simulink model "pmdc_simulink"  (R2025b)
settings: Solver=VariableStepAuto  StartTime=0.0  StopTime=3  RelTol=1e-3
undefined symbols (not defined in the file or in its folder): Bm, J, Kv, La, Ra, TL, Va
settings Model: Creator=Seyma  LastModifiedBy=Seyma
settings DataIOCC: SaveFormat=Array  ReturnWorkspaceOutputs=off

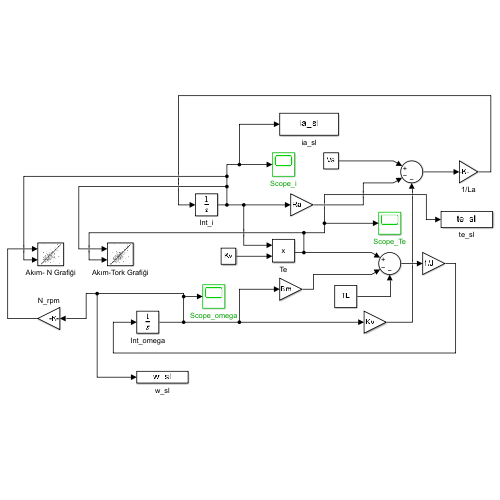
[thumbnail: Simulink's stored preview of the top-level diagram]
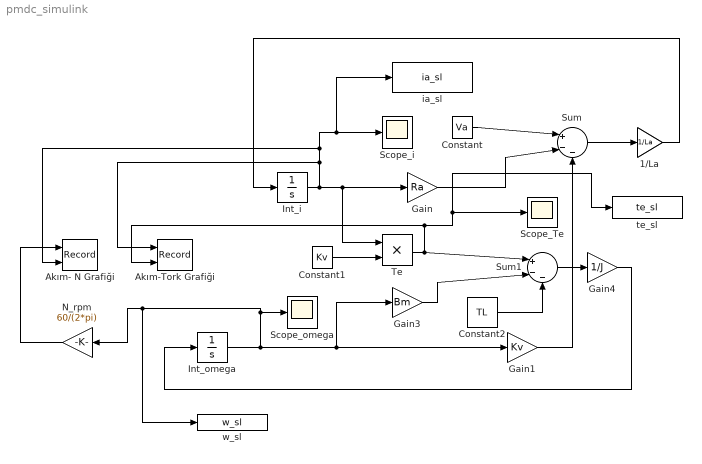
== system pmdc_simulink ==
  1/La : Gain  Gain=1/La
  Akım- N Grafiği : Record  NumPorts=2.0  FileSettingsInternal="{\"entries\":[{\"content\":{\"excelSettings\":{\"content\":{},\"type\":\"Streamout.ExcelSettings\"},\"parquetSettings\":{\"content\":{},\"type\":\"Streamout.ParquetSettings\"}},\"type\":\"Streamout.FileSettingStorage\",\"uuid\":\"\"}],\"packageUris\":[\"http:\\/\\/schema.mathworks.com\\/mf0\\/streamout_blocks\\/R2020a\"],\"version\":\"1.0\"}"  FrameSettings=[0, 0]  Layout=[1 1]  SignalsInternal="{\"entries\":[{\"content\":{\"signals\":[{\"content\":{\"blockPath\":[],\"dimensions\":[1],\"domain\":\"\",\"lineColor\":\"#a2142f\",\"lineWidth\":2,\"plots\":[ 1 ],\"port\":1,\"sid\":[\"\"],\"signalID\":1,\"signalName\":\"N_rpm\"},\"type\":\"RecordBlkView.Signal\",\"uuid\":\"\"},{\"content\":{\"blockPath\":[],\"dimensions\":[1],\"domain\":\"\",\"lineColor\":\"#139fff\",\"lineWidth\":2,\"plots\":[ 1 ],\"port\":2,\"sid\":[\"\"],\"signalID\":2,\"signalName\":\"Int_i\"},\"type\":\"RecordBlkView.Signal\",\"uuid\":\"\"}]},\"type\":\"RecordBlkView.InputSignals\",\"uuid\":\"\"}],\"packageUris\":[\"http:\\/\\/schema.mathworks.com\\/mf0\\/streamout_blocks\\/R2020a\"],\"version\":\"1.0\"}"  VisualizationBindings="{\"xyplotplugin\":{\"info\":[{\"series\":[{\"bindingParametersList\":[{\"parameter\":\"X-Axis\",\"signalID\":2,\"signalName\":\"Int_i\"},{\"parameter\":\"Y-Axis\",\"signalID\":1,\"signalName\":\"N_rpm\"}],\"seriesID\":0}],\"subplotID\":1}]}}"  CompatibilityTag=XY
  Akım-Tork Grafiği : Record  NumPorts=2.0  FileSettingsInternal="{\"entries\":[{\"content\":{\"excelSettings\":{\"content\":{},\"type\":\"Streamout.ExcelSettings\"},\"parquetSettings\":{\"content\":{},\"type\":\"Streamout.ParquetSettings\"}},\"type\":\"Streamout.FileSettingStorage\",\"uuid\":\"\"}],\"packageUris\":[\"http:\\/\\/schema.mathworks.com\\/mf0\\/streamout_blocks\\/R2020a\"],\"version\":\"1.0\"}"  FrameSettings=[0, 0]  Layout=[1 1]  SignalsInternal="{\"entries\":[{\"content\":{\"signals\":[{\"content\":{\"blockPath\":[],\"dimensions\":[1],\"domain\":\"\",\"lineColor\":\"#a2142f\",\"plots\":[ 1 ],\"port\":1,\"sid\":[\"\"],\"signalID\":1,\"signalName\":\"Int_i\"},\"type\":\"RecordBlkView.Signal\",\"uuid\":\"\"},{\"content\":{\"blockPath\":[],\"dimensions\":[1],\"domain\":\"\",\"lineColor\":\"#139fff\",\"plots\":[ 1 ],\"port\":2,\"sid\":[\"\"],\"signalID\":2,\"signalName\":\"Te\"},\"type\":\"RecordBlkView.Signal\",\"uuid\":\"\"}]},\"type\":\"RecordBlkView.InputSignals\",\"uuid\":\"\"}],\"packageUris\":[\"http:\\/\\/schema.mathworks.com\\/mf0\\/streamout_blocks\\/R2020a\"],\"version\":\"1.0\"}"  VisualizationBindings="{\"xyplotplugin\":{\"info\":[{\"series\":[{\"bindingParametersList\":[{\"parameter\":\"X-Axis\",\"signalID\":2,\"signalName\":\"Te\"},{\"parameter\":\"Y-Axis\",\"signalID\":1,\"signalName\":\"Int_i\"}],\"seriesID\":0}],\"subplotID\":1}]}}"  CompatibilityTag=XY
  Constant : Constant  Value=Va
  Constant1 : Constant  Value=Kv
  Constant2 : Constant  Value=TL
  Gain : Gain  Gain=Ra
  Gain1 : Gain  Gain=Kv
  Gain3 : Gain  Gain=Bm
  Gain4 : Gain  Gain=1/J
  Int_i : Integrator
  Int_omega : Integrator
  N_rpm : Gain  Gain=60/(2*pi)
  Scope_Te : Scope
      settings: ActiveDisplayYMinimum=-1  ActiveDisplayYMaximum=1  DataLoggingVariableName=ScopeData2
  Scope_i : Scope
      settings: ActiveDisplayYMinimum=-1  ActiveDisplayYMaximum=1
  Scope_omega : Scope
      settings: ActiveDisplayYMinimum=-36.424268325134172  ActiveDisplayYMaximum=298.05342921303554
  Sum : Sum  Inputs=|+--
  Sum1 : Sum  Inputs=|+--
  Te : Product
  "ia_sl " : ToWorkspace  VariableName=ia_sl  SampleTime=-1
  "te_sl " : ToWorkspace  VariableName=te_sl  SampleTime=-1
  "w_sl " : ToWorkspace  VariableName=w_sl  SampleTime=-1
  wires:
  Constant/1 -> Sum/1
  Gain/1 -> Sum/2
  Int_omega/1 -> N_rpm/1, "w_sl "/1, Scope_omega/1, Gain1/1, Gain3/1
  Gain1/1 -> Sum/3
  Sum/1 -> 1/La/1
  1/La/1 -> Int_i/1
  Constant1/1 -> Te/2
  Te/1 -> Akım-Tork Grafiği/2, "te_sl "/1, Scope_Te/1, Sum1/1
  Gain3/1 -> Sum1/2
  Constant2/1 -> Sum1/3
  Sum1/1 -> Gain4/1
  Gain4/1 -> Int_omega/1
  Int_i/1 -> "ia_sl "/1, Scope_i/1, Akım- N Grafiği/2, Akım-Tork Grafiği/1, Te/1, Gain/1
  N_rpm/1 -> Akım- N Grafiği/1
